simulink model "impedance_control"  (R2021b)
settings: Solver=FixedStepAuto  StartTime=0.0  StopTime=10  FixedStep=Ts  RelTol=1e-3
undefined symbols (not defined in the file): dqi, invMd, K, KD, KP, Md, myRobot, qi, qr, xr
settings Model: Creator=simon  LastModifiedBy=miche
settings SolverCC: ZeroCrossControl=DisableAll  AlgebraicLoopSolver=TrustRegion
settings DebuggingCC: SFMachineParentedDataDiag=warning

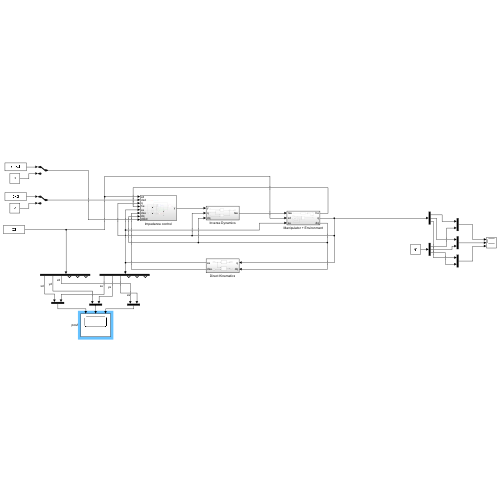
[thumbnail: Simulink's stored preview of the top-level diagram]
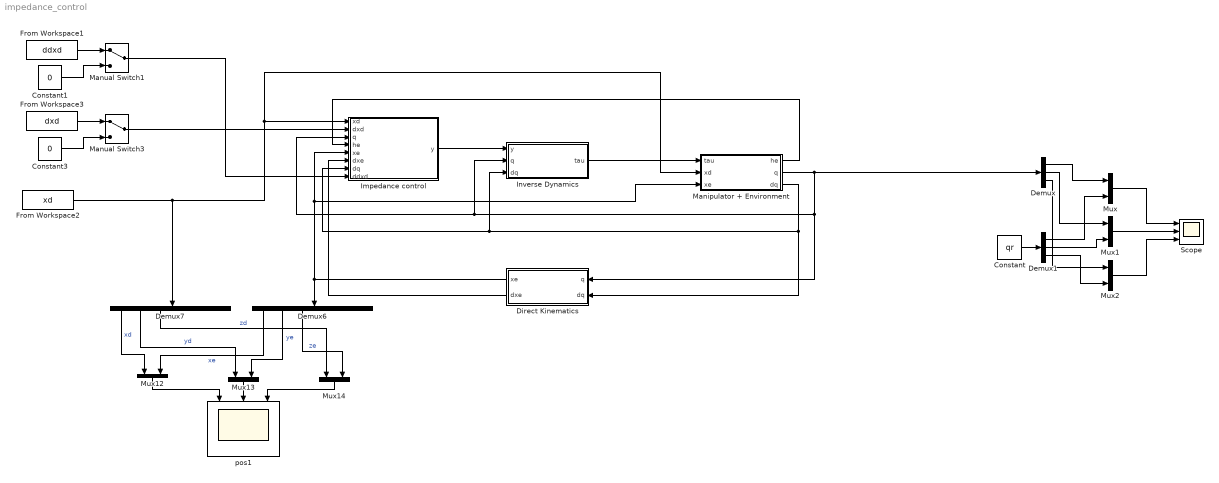
== system impedance_control ==
  Constant : Constant  Value=qr
  Constant1 : Constant  Value=0
  Constant3 : Constant  Value=0
  Demux : Demux  Outputs=3
  Demux1 : Demux  Outputs=3
  Demux6 : Demux  Outputs=6
  Demux7 : Demux  Outputs=6
  Direct Kinematics : Subsystem
  From Workspace1 : FromWorkspace  VariableName=ddxd
  From Workspace2 : FromWorkspace  VariableName=xd
  From Workspace3 : FromWorkspace  VariableName=dxd
  Impedance control : Subsystem
  Inverse Dynamics : Subsystem
  Manipulator + Environment : Subsystem
  Manual Switch1 : ManualSwitch
  Manual Switch3 : ManualSwitch
  Mux{,1..2,12..14} (6 alike) : Mux  Inputs=2
  Scope : Scope  NumInputPorts=3
  pos1 : Scope  NumInputPorts=3
  wires:
  Direct Kinematics/2(dxe) -> Impedance control/6(dxe)
  Impedance control/1(y) -> Inverse Dynamics/1(y)
  Inverse Dynamics/1(tau) -> Manipulator + Environment/1(tau)
  Manipulator + Environment/2(q) -> Inverse Dynamics/2(q), Impedance control/3(q), Direct Kinematics/1(q), Demux/1
  Manipulator + Environment/3(dq) -> Direct Kinematics/2(dq), Impedance control/7(dq), Inverse Dynamics/3(dq)
  Manipulator + Environment/1(he) -> Impedance control/4(he)
  From Workspace3/1 -> Manual Switch3/1
  Constant3/1 -> Manual Switch3/2
  Manual Switch3/1 -> Impedance control/2(dxd)
  Demux7/3 -> Mux14/1  "zd"
  Direct Kinematics/1(xe) -> Demux6/1, Impedance control/5(xe), Manipulator + Environment/3(xe)
  From Workspace2/1 -> Impedance control/1(xd), Manipulator + Environment/2(xd), Demux7/1
  Demux7/2 -> Mux13/1  "yd"
  Mux14/1 -> pos1/3
  Demux7/1 -> Mux12/1  "xd"
  Demux6/2 -> Mux13/2  "ye"
  Demux6/1 -> Mux12/2  "xe"
  Demux6/3 -> Mux14/2  "ze"
  Mux12/1 -> pos1/1
  Mux13/1 -> pos1/2
  Constant1/1 -> Manual Switch1/2
  From Workspace1/1 -> Manual Switch1/1
  Manual Switch1/1 -> Impedance control/8(ddxd)
  Demux/1 -> Mux/1
  Constant/1 -> Demux1/1
  Demux/2 -> Mux1/1
  Demux/3 -> Mux2/1
  Demux1/1 -> Mux/2
  Demux1/2 -> Mux1/2
  Demux1/3 -> Mux2/2
  Mux/1 -> Scope/1
  Mux1/1 -> Scope/2
  Mux2/1 -> Scope/3

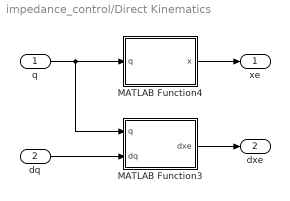
== system impedance_control/Direct Kinematics ==
  q : Inport
  dq : Inport  Port=2
  MATLAB Function3 : MATLAB Function  TreatAsAtomicUnit=on
  MATLAB Function4 : MATLAB Function  TreatAsAtomicUnit=on
  xe : Outport
  dxe : Outport  Port=2
  wires:
  MATLAB Function3/1(dxe) -> dxe/1
  dq/1 -> MATLAB Function3/2(dq)
  q/1 -> MATLAB Function3/1(q), MATLAB Function4/1(q)
  MATLAB Function4/1(x) -> xe/1

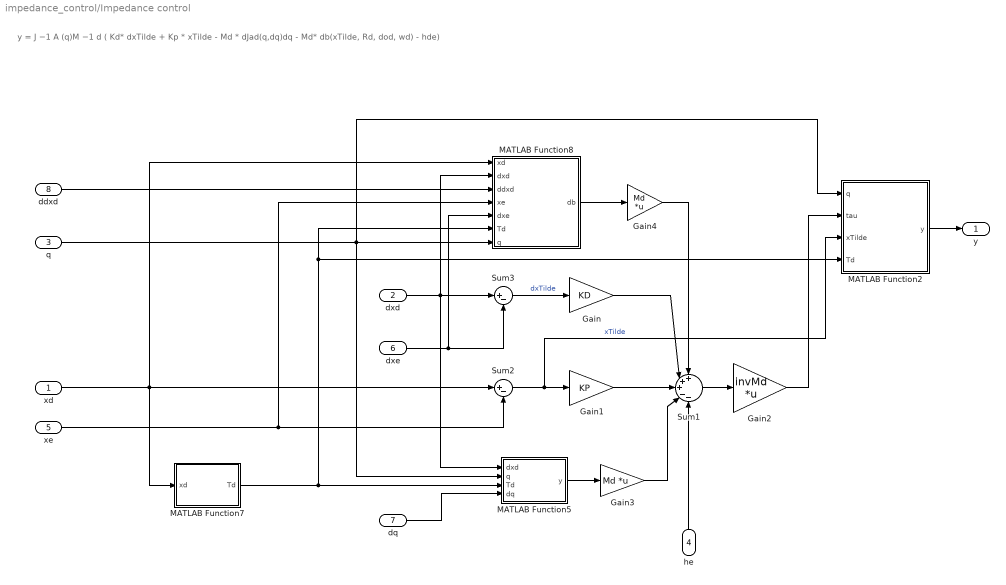
== system impedance_control/Impedance control ==
  note: y = J −1 A (q)M −1 d ( Kd* dxTilde + Kp * xTilde - Md * dJad(q,dq)dq - Md* db(xTilde, Rd, dod, wd) - hde)
  xd : Inport
  dxd : Inport  Port=2
  q : Inport  Port=3
  he : Inport  Port=4
  xe : Inport  Port=5
  dxe : Inport  Port=6
  dq : Inport  Port=7
  ddxd : Inport  Port=8
  Gain : Gain  Gain=KD
  Gain1 : Gain  Gain=KP
  Gain2 : Gain  Gain=invMd  Multiplication=Matrix(K*u)
  Gain3 : Gain  Gain=Md  Multiplication=Matrix(K*u)
  Gain4 : Gain  Gain=Md  Multiplication=Matrix(K*u)
  MATLAB Function2 : MATLAB Function  TreatAsAtomicUnit=on
  MATLAB Function5 : MATLAB Function  TreatAsAtomicUnit=on
  MATLAB Function7 : MATLAB Function  TreatAsAtomicUnit=on
  MATLAB Function8 : MATLAB Function  TreatAsAtomicUnit=on
  Sum1 : Sum  Inputs=+++--
  Sum2 : Sum  Inputs=|+-
  Sum3 : Sum  Inputs=|+-
  y : Outport
  wires:
  MATLAB Function7/1(Td) -> MATLAB Function5/3(Td), MATLAB Function2/4(Td), MATLAB Function8/6(Td)
  MATLAB Function8/1(db) -> Gain4/1
  MATLAB Function5/1(y) -> Gain3/1
  Gain2/1 -> MATLAB Function2/2(tau)
  dxd/1 -> MATLAB Function8/2(dxd), MATLAB Function5/1(dxd), Sum3/1
  xd/1 -> MATLAB Function8/1(xd), MATLAB Function7/1(xd), Sum2/1
  Gain3/1 -> Sum1/4
  MATLAB Function2/1(y) -> y/1
  Gain/1 -> Sum1/2
  Sum3/1 -> Gain/1  "dxTilde"
  Sum1/1 -> Gain2/1
  Gain1/1 -> Sum1/3
  Gain4/1 -> Sum1/1
  q/1 -> MATLAB Function2/1(q), MATLAB Function5/2(q), MATLAB Function8/7(q)
  xe/1 -> MATLAB Function8/4(xe), Sum2/2
  dxe/1 -> Sum3/2, MATLAB Function8/5(dxe)
  dq/1 -> MATLAB Function5/4(dq)
  ddxd/1 -> MATLAB Function8/3(ddxd)
  Sum2/1 -> MATLAB Function2/3(xTilde), Gain1/1  "xTilde"
  he/1 -> Sum1/5

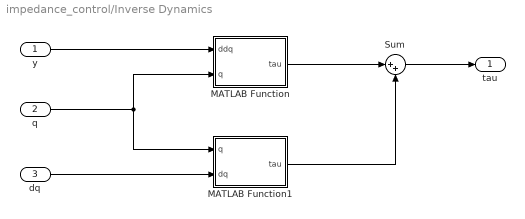
== system impedance_control/Inverse Dynamics ==
  y : Inport
  q : Inport  Port=2
  dq : Inport  Port=3
  MATLAB Function : MATLAB Function  TreatAsAtomicUnit=on
  MATLAB Function1 : MATLAB Function  TreatAsAtomicUnit=on
  Sum : Sum  Inputs=|++
  tau : Outport
  wires:
  MATLAB Function1/1(tau) -> Sum/2
  MATLAB Function/1(tau) -> Sum/1
  y/1 -> MATLAB Function/1(ddq)
  Sum/1 -> tau/1
  dq/1 -> MATLAB Function1/2(dq)
  q/1 -> MATLAB Function/2(q), MATLAB Function1/1(q)

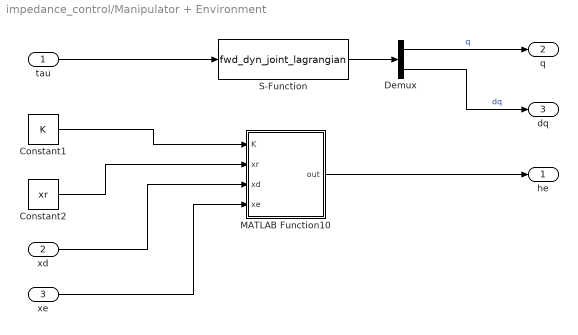
== system impedance_control/Manipulator + Environment ==
  tau : Inport
  xd : Inport  Port=2
  xe : Inport  Port=3
  Constant1 : Constant  Value=K
  Constant2 : Constant  Value=xr
  Demux : Demux  Outputs=2
  MATLAB Function10 : MATLAB Function  TreatAsAtomicUnit=on
  S-Function : S-Function  FunctionName=fwd_dyn_joint_lagrangian  Parameters=myRobot,qi,dqi  SFunctionDeploymentMode=off  EnableBusSupport=off
  he : Outport
  q : Outport  Port=2
  dq : Outport  Port=3
  wires:
  tau/1 -> S-Function/1
  Constant1/1 -> MATLAB Function10/1(K)
  Constant2/1 -> MATLAB Function10/2(xr)
  xd/1 -> MATLAB Function10/3(xd)
  xe/1 -> MATLAB Function10/4(xe)
  S-Function/1 -> Demux/1
  Demux/1 -> q/1  "q"
  Demux/2 -> dq/1  "dq"
  MATLAB Function10/1(out) -> he/1

== matlab function impedance_control/Direct Kinematics/MATLAB Function3 ==
  data: q input; dxe output; dq input
function dxe = Ja(q, dq)

dxe = getJa(q)*dq;

== matlab function impedance_control/Impedance control/MATLAB Function2 ==
  data: q input; y output; tau input; xTilde input; Td input
function y = invJad(q, tau, xTilde, Td)
jad = getJad(q, xTilde, Td);
y = pinv(jad)*tau;

== matlab function impedance_control/Direct Kinematics/MATLAB Function4 ==
  data: q input; x output
function x = k(q)

x = getK(q);

== matlab function impedance_control/Impedance control/MATLAB Function5 ==
  data: dxd input; q input; Td input; y output; dq input
function y = dJadq(dxd, q, Td,dq)
    y = getDiffJad(dxd,q,Td,dq)*dq;

== matlab function impedance_control/Impedance control/MATLAB Function7 ==
  data: xd input; Td output
function Td = getTd(xd)
Rd = eul2rotm(xd(4:6)','ZYZ');
t = xd(1:3);
Td = [Rd t
    zeros(1,3) 1];

== matlab function impedance_control/Impedance control/MATLAB Function8 ==
  data: xd input; dxd input; ddxd input; xe input; dxe input; db output; Td input; q input
function db = diffB(xd,dxd,ddxd,xe,dxe, Td,q)

db = getDiffImpB(xd,dxd,ddxd,xe,dxe, Td,q);

== matlab function impedance_control/Inverse Dynamics/MATLAB Function ==
  data: ddq input size=3; q input size=3; tau output
function tau = B(ddq,q) 

tau = getB(q)*ddq;

== matlab function impedance_control/Inverse Dynamics/MATLAB Function1 ==
  data: q input size=3; tau output; dq input size=3
function tau = n(q, dq)

tau = getN(q, dq);

== matlab function impedance_control/Manipulator + Environment/MATLAB Function10 ==
  data: K input; out output size=6; xr input; xd input; xe input size=6
function out = hde(K,xr, xd, xe)
%consider the interaction only in z direction
if xe(3) < xr(3)
    dxrd = xd-xr;
    dxed = xd-xe;
    dxre = dxrd-dxed;
    he = K*dxre;
else
    he = zeros(6,1);
end

out = he;
